simulink model "WInd_Blade_Simulation"  (R2022b)
settings: Solver=VariableStepAuto  StartTime=0.0  StopTime=10.0  RelTol=1e-3
settings Model: Creator=jayesh sunil gurav  LastModifiedBy=Amol Gavit
settings DebuggingCC: UnconnectedInputMsg=warning  UnconnectedOutputMsg=warning  UnconnectedLineMsg=warning
settings ModelReferenceCC: EnableRefExpFcnMdlSchedulingChecks=on
settings RTWCC: DLArmComputeVersion=19.05

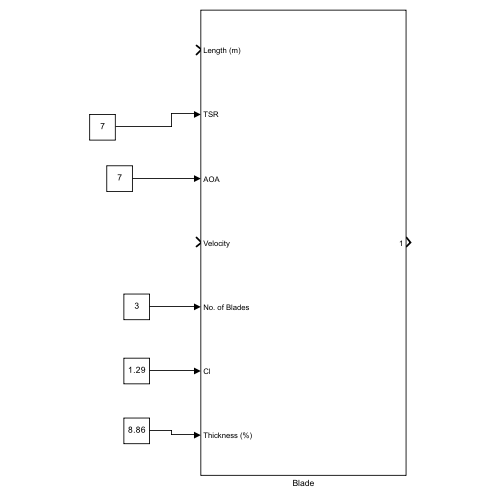
[thumbnail: Simulink's stored preview of the top-level diagram]
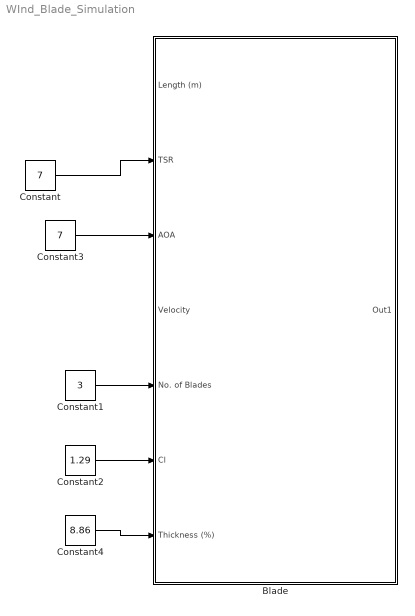
== system WInd_Blade_Simulation ==
  Blade : Subsystem
  Constant : Constant  Value=7
  Constant1 : Constant  Value=3
  Constant2 : Constant  Value=1.29
  Constant3 : Constant  Value=7
  Constant4 : Constant  Value=8.86
  wires:
  Constant/1 -> Blade/2(TSR)
  Constant1/1 -> Blade/5(No. of Blades)
  Constant2/1 -> Blade/6(Cl)
  Constant3/1 -> Blade/3(AOA)
  Constant4/1 -> Blade/7(Thickness (%))

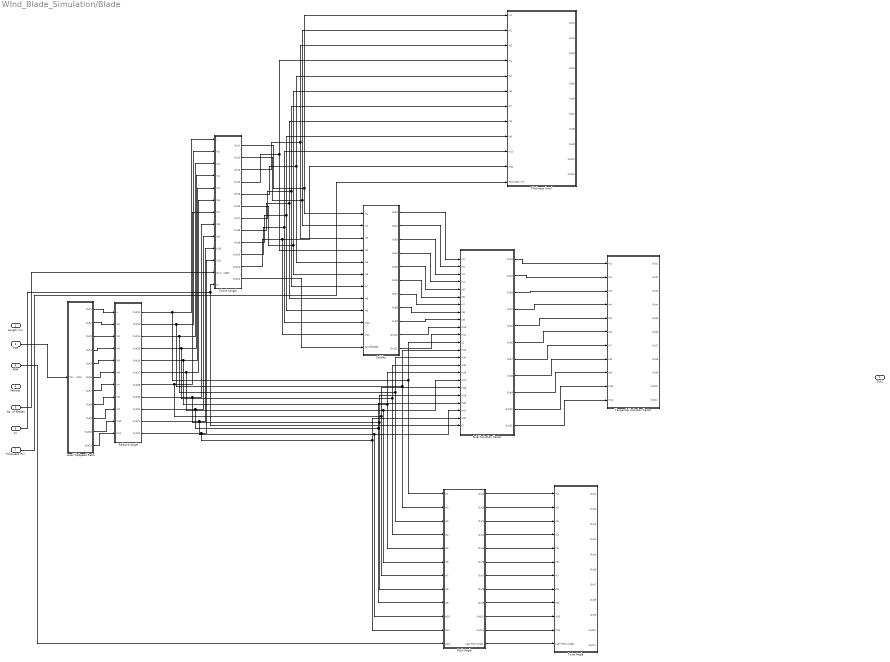
== system WInd_Blade_Simulation/Blade ==
  Length (m) : Inport
  TSR : Inport  Port=2
  AOA : Inport  Port=3
  Velocity : Inport  Port=4
  No. of Blades : Inport  Port=5
  Cl : Inport  Port=6
  Thickness (%) : Inport  Port=7
  Axial Induction Factor : Subsystem
  Chord Length : Subsystem
  Local TipSpeed Ratio : Subsystem
  Pitch Angle : Subsystem
  Relative Angle : Subsystem
  Solidity : Subsystem
  Tangential Induction Factor : Subsystem
  Thickness (mm) : Subsystem
  Twist Angle : Subsystem
  Out1 : Outport
  wires:
  TSR/1 -> Local TipSpeed Ratio/1(Tip Speed ratio)
  Local TipSpeed Ratio/1(Out1) -> Relative Angle/1(u)
  Local TipSpeed Ratio/2(Out2) -> Relative Angle/2(In2)
  Local TipSpeed Ratio/11(Out11) -> Relative Angle/11(In11)
  Local TipSpeed Ratio/10(Out10) -> Relative Angle/10(In10)
  Local TipSpeed Ratio/9(Out9) -> Relative Angle/9(In9)
  Local TipSpeed Ratio/8(Out8) -> Relative Angle/8(In8)
  Local TipSpeed Ratio/7(Out7) -> Relative Angle/7(In7)
  Local TipSpeed Ratio/6(Out6) -> Relative Angle/6(In6)
  Local TipSpeed Ratio/5(Out5) -> Relative Angle/5(In5)
  Local TipSpeed Ratio/4(Out4) -> Relative Angle/4(In4)
  Local TipSpeed Ratio/3(Out3) -> Relative Angle/3(In3)
  Relative Angle/1(Out12) -> Pitch Angle/1(In1), Axial Induction Factor/12(12), Chord Length/1(1)
  Relative Angle/2(Out13) -> Pitch Angle/2(In2), Axial Induction Factor/13(In13), Chord Length/2(In2)
  Relative Angle/3(Out14) -> Pitch Angle/3(In3), Axial Induction Factor/14(In14), Chord Length/3(In3)
  Relative Angle/4(Out15) -> Pitch Angle/4(In4), Axial Induction Factor/15(In15), Chord Length/4(In4)
  Relative Angle/5(Out16) -> Pitch Angle/5(In5), Axial Induction Factor/16(In16), Chord Length/5(In5)
  Relative Angle/6(Out17) -> Pitch Angle/6(In6), Axial Induction Factor/17(In17), Chord Length/6(In6)
  Relative Angle/7(Out18) -> Pitch Angle/7(In7), Axial Induction Factor/18(In18), Chord Length/7(In7)
  Relative Angle/8(Out19) -> Pitch Angle/8(In8), Axial Induction Factor/19(In19), Chord Length/8(In8)
  Relative Angle/9(Out20) -> Pitch Angle/9(In9), Axial Induction Factor/20(In20), Chord Length/9(In9)
  Relative Angle/10(Out21) -> Pitch Angle/10(In10), Axial Induction Factor/21(In21), Chord Length/10(In10)
  Relative Angle/11(Out22) -> Pitch Angle/11(In11), Axial Induction Factor/22(In22), Chord Length/11(In11)
  No. of Blades/1 -> Chord Length/12(No of Blades)
  Cl/1 -> Chord Length/13(Cl), Axial Induction Factor/23(Cl)
  Chord Length/2(Out2) -> Thickness (mm)/2(In2), Solidity/2(In2)
  Chord Length/3(Out3) -> Solidity/3(In3), Thickness (mm)/3(In3)
  Chord Length/4(Out4) -> Solidity/4(In4), Thickness (mm)/4(In4)
  Chord Length/5(Out5) -> Solidity/5(In5), Thickness (mm)/5(In5)
  Chord Length/6(Out6) -> Solidity/6(In6), Thickness (mm)/6(In6)
  Chord Length/7(Out7) -> Solidity/7(In7), Thickness (mm)/7(In7)
  Chord Length/8(Out8) -> Solidity/8(In8), Thickness (mm)/8(In8)
  Chord Length/9(Out9) -> Solidity/9(In9), Thickness (mm)/9(In9)
  Chord Length/10(Out10) -> Solidity/10(In10), Thickness (mm)/10(In12)
  Chord Length/11(Out11) -> Solidity/11(In11), Thickness (mm)/11(In10)
  Chord Length/12(Out12) -> Solidity/12(No of Blades)
  Solidity/1(Out1) -> Axial Induction Factor/1(In1)
  Solidity/2(Out2) -> Axial Induction Factor/2(In2)
  Solidity/3(Out3) -> Axial Induction Factor/3(In3)
  Solidity/4(Out4) -> Axial Induction Factor/4(In4)
  Solidity/5(Out5) -> Axial Induction Factor/5(In5)
  Solidity/6(Out6) -> Axial Induction Factor/6(In6)
  Solidity/7(Out7) -> Axial Induction Factor/7(In7)
  Solidity/8(Out8) -> Axial Induction Factor/8(In8)
  Solidity/9(Out9) -> Axial Induction Factor/9(In9)
  Solidity/10(Out10) -> Axial Induction Factor/10(In10)
  Solidity/11(Out11) -> Axial Induction Factor/11(In11)
  Axial Induction Factor/1(Out1) -> Tangential Induction Factor/1(In1)
  Axial Induction Factor/2(Out2) -> Tangential Induction Factor/2(In2)
  Axial Induction Factor/3(Out3) -> Tangential Induction Factor/3(In3)
  Axial Induction Factor/4(Out4) -> Tangential Induction Factor/4(In4)
  Axial Induction Factor/5(Out5) -> Tangential Induction Factor/5(In5)
  Axial Induction Factor/6(Out6) -> Tangential Induction Factor/6(In6)
  Axial Induction Factor/7(Out7) -> Tangential Induction Factor/7(In7)
  Axial Induction Factor/8(Out8) -> Tangential Induction Factor/8(In8)
  Axial Induction Factor/9(Out9) -> Tangential Induction Factor/9(In9)
  Axial Induction Factor/10(Out10) -> Tangential Induction Factor/10(In10)
  Axial Induction Factor/11(Out11) -> Tangential Induction Factor/11(In11)
  AOA/1 -> Pitch Angle/12(AOA)
  Pitch Angle/1(Out1) -> Twist Angle/1(In1)
  Pitch Angle/2(Out3) -> Twist Angle/2(In2)
  Pitch Angle/3(Out2) -> Twist Angle/3(In3)
  Pitch Angle/4(Out4) -> Twist Angle/4(In4)
  Pitch Angle/5(Out5) -> Twist Angle/5(In5)
  Pitch Angle/6(Out6) -> Twist Angle/6(In6)
  Pitch Angle/7(Out7) -> Twist Angle/7(In7)
  Pitch Angle/8(Out8) -> Twist Angle/8(In8)
  Pitch Angle/9(Out9) -> Twist Angle/9(In9)
  Pitch Angle/10(Out10) -> Twist Angle/10(In10)
  Pitch Angle/11(Out11) -> Twist Angle/11(In11)
  Pitch Angle/12(Last Pitch angle) -> Twist Angle/12(Last Pitch Anlge)
  Chord Length/1(Out1) -> Thickness (mm)/1(In1), Solidity/1(In1)
  Thickness (%)/1 -> Thickness (mm)/12(Thickness (%))

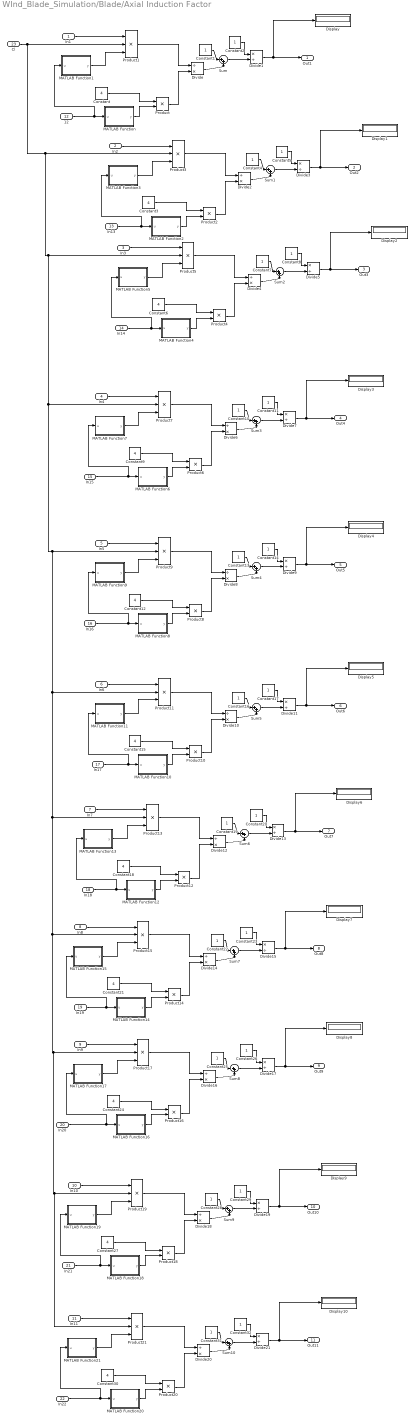
== system WInd_Blade_Simulation/Blade/Axial Induction Factor ==
  In1 : Inport
  In2 : Inport  Port=2
  In3 : Inport  Port=3
  In4 : Inport  Port=4
  In5 : Inport  Port=5
  In6 : Inport  Port=6
  In7 : Inport  Port=7
  In8 : Inport  Port=8
  In9 : Inport  Port=9
  In10 : Inport  Port=10
  In11 : Inport  Port=11
  12 : Inport  Port=12
  In13 : Inport  Port=13
  In14 : Inport  Port=14
  In15 : Inport  Port=15
  In16 : Inport  Port=16
  In17 : Inport  Port=17
  In18 : Inport  Port=18
  In19 : Inport  Port=19
  In20 : Inport  Port=20
  In21 : Inport  Port=21
  In22 : Inport  Port=22
  Cl : Inport  Port=23
  Constant{,3,6,9,12,15,18,21,24,27,30} (11 alike) : Constant  Value=4
  Constant{1..2,4..5,7..8,10..11,13..14,16..17,19..20,22..23,25..26,28..29,31..32} (22 alike) : Constant
  Display{,1..10} (11 alike) : Display
  Divide{,2,4,6,8,10,12,14,16,18,20} (11 alike) : Product  Inputs=/*
  Divide{1,3,5,7,9,11,13,15,17,19,21} (11 alike) : Product  Inputs=*/
  MATLAB Function : MATLAB Function  TreatAsAtomicUnit=on
  MATLAB Function1 : MATLAB Function  TreatAsAtomicUnit=on
  MATLAB Function10 : MATLAB Function  TreatAsAtomicUnit=on
  MATLAB Function11 : MATLAB Function  TreatAsAtomicUnit=on
  MATLAB Function12 : MATLAB Function  TreatAsAtomicUnit=on
  MATLAB Function13 : MATLAB Function  TreatAsAtomicUnit=on
  MATLAB Function14 : MATLAB Function  TreatAsAtomicUnit=on
  MATLAB Function15 : MATLAB Function  TreatAsAtomicUnit=on
  MATLAB Function16 : MATLAB Function  TreatAsAtomicUnit=on
  MATLAB Function17 : MATLAB Function  TreatAsAtomicUnit=on
  MATLAB Function18 : MATLAB Function  TreatAsAtomicUnit=on
  MATLAB Function19 : MATLAB Function  TreatAsAtomicUnit=on
  MATLAB Function2 : MATLAB Function  TreatAsAtomicUnit=on
  MATLAB Function20 : MATLAB Function  TreatAsAtomicUnit=on
  MATLAB Function21 : MATLAB Function  TreatAsAtomicUnit=on
  MATLAB Function3 : MATLAB Function  TreatAsAtomicUnit=on
  MATLAB Function4 : MATLAB Function  TreatAsAtomicUnit=on
  MATLAB Function5 : MATLAB Function  TreatAsAtomicUnit=on
  MATLAB Function6 : MATLAB Function  TreatAsAtomicUnit=on
  MATLAB Function7 : MATLAB Function  TreatAsAtomicUnit=on
  MATLAB Function8 : MATLAB Function  TreatAsAtomicUnit=on
  MATLAB Function9 : MATLAB Function  TreatAsAtomicUnit=on
  Product{,2,4,6,8,10,12,14,16,18,20} (11 alike) : Product
  Product{1,3,5,7,9,11,13,15,17,19,21} (11 alike) : Product  Inputs=3
  Sum{,1..10} (11 alike) : Sum  Inputs=|++
  Out1 : Outport
  Out2 : Outport  Port=2
  Out3 : Outport  Port=3
  Out4 : Outport  Port=4
  Out5 : Outport  Port=5
  Out6 : Outport  Port=6
  Out7 : Outport  Port=7
  Out8 : Outport  Port=8
  Out9 : Outport  Port=9
  Out10 : Outport  Port=10
  Out11 : Outport  Port=11
  wires:
  Constant/1 -> Product/1
  12/1 -> MATLAB Function1/1(u), MATLAB Function/1(u)
  MATLAB Function/1(y) -> Product/2
  In1/1 -> Product1/1
  MATLAB Function1/1(y) -> Product1/3
  Product1/1 -> Divide/1
  Product/1 -> Divide/2
  Constant1/1 -> Sum/1
  Divide/1 -> Sum/2
  Sum/1 -> Divide1/2
  Constant2/1 -> Divide1/1
  Divide1/1 -> Display/1, Out1/1
  In13/1 -> MATLAB Function2/1(u), MATLAB Function3/1(u)
  Sum1/1 -> Divide3/2
  MATLAB Function3/1(y) -> Product3/3
  Divide2/1 -> Sum1/2
  Divide3/1 -> Display1/1, Out2/1
  Product3/1 -> Divide2/1
  In2/1 -> Product3/1
  MATLAB Function2/1(y) -> Product2/2
  Constant4/1 -> Sum1/1
  Constant3/1 -> Product2/1
  Constant5/1 -> Divide3/1
  Product2/1 -> Divide2/2
  In14/1 -> MATLAB Function5/1(u), MATLAB Function4/1(u)
  Sum2/1 -> Divide5/2
  MATLAB Function5/1(y) -> Product5/3
  Divide4/1 -> Sum2/2
  Divide5/1 -> Display2/1, Out3/1
  Product5/1 -> Divide4/1
  In3/1 -> Product5/1
  MATLAB Function4/1(y) -> Product4/2
  Constant7/1 -> Sum2/1
  Constant6/1 -> Product4/1
  Constant8/1 -> Divide5/1
  Product4/1 -> Divide4/2
  In15/1 -> MATLAB Function7/1(u), MATLAB Function6/1(u)
  Sum3/1 -> Divide7/2
  MATLAB Function7/1(y) -> Product7/3
  Divide6/1 -> Sum3/2
  Divide7/1 -> Display3/1, Out4/1
  Product7/1 -> Divide6/1
  In4/1 -> Product7/1
  MATLAB Function6/1(y) -> Product6/2
  Constant10/1 -> Sum3/1
  Constant9/1 -> Product6/1
  Constant11/1 -> Divide7/1
  Product6/1 -> Divide6/2
  In16/1 -> MATLAB Function9/1(u), MATLAB Function8/1(u)
  Sum4/1 -> Divide9/2
  MATLAB Function9/1(y) -> Product9/3
  Divide8/1 -> Sum4/2
  Divide9/1 -> Display4/1, Out5/1
  Product9/1 -> Divide8/1
  In5/1 -> Product9/1
  MATLAB Function8/1(y) -> Product8/2
  Constant13/1 -> Sum4/1
  Constant12/1 -> Product8/1
  Constant14/1 -> Divide9/1
  Product8/1 -> Divide8/2
  In17/1 -> MATLAB Function11/1(u), MATLAB Function10/1(u)
  Sum5/1 -> Divide11/2
  MATLAB Function11/1(y) -> Product11/3
  Divide10/1 -> Sum5/2
  Divide11/1 -> Display5/1, Out6/1
  Product11/1 -> Divide10/1
  In6/1 -> Product11/1
  MATLAB Function10/1(y) -> Product10/2
  Constant16/1 -> Sum5/1
  Constant15/1 -> Product10/1
  Constant17/1 -> Divide11/1
  Product10/1 -> Divide10/2
  In18/1 -> MATLAB Function13/1(u), MATLAB Function12/1(u)
  Sum6/1 -> Divide13/2
  MATLAB Function13/1(y) -> Product13/3
  Divide12/1 -> Sum6/2
  Divide13/1 -> Display6/1, Out7/1
  Product13/1 -> Divide12/1
  In7/1 -> Product13/1
  MATLAB Function12/1(y) -> Product12/2
  Constant19/1 -> Sum6/1
  Constant18/1 -> Product12/1
  Constant20/1 -> Divide13/1
  Product12/1 -> Divide12/2
  In19/1 -> MATLAB Function14/1(u), MATLAB Function15/1(u)
  Sum7/1 -> Divide15/2
  MATLAB Function15/1(y) -> Product15/3
  Divide14/1 -> Sum7/2
  Divide15/1 -> Display7/1, Out8/1
  Product15/1 -> Divide14/1
  In8/1 -> Product15/1
  MATLAB Function14/1(y) -> Product14/2
  Constant22/1 -> Sum7/1
  Constant21/1 -> Product14/1
  Constant23/1 -> Divide15/1
  Product14/1 -> Divide14/2
  In20/1 -> MATLAB Function17/1(u), MATLAB Function16/1(u)
  Sum8/1 -> Divide17/2
  MATLAB Function17/1(y) -> Product17/3
  Divide16/1 -> Sum8/2
  Divide17/1 -> Display8/1, Out9/1
  Product17/1 -> Divide16/1
  In9/1 -> Product17/1
  MATLAB Function16/1(y) -> Product16/2
  Constant25/1 -> Sum8/1
  Constant24/1 -> Product16/1
  Constant26/1 -> Divide17/1
  Product16/1 -> Divide16/2
  In21/1 -> MATLAB Function19/1(u), MATLAB Function18/1(u)
  Sum9/1 -> Divide19/2
  MATLAB Function19/1(y) -> Product19/3
  Divide18/1 -> Sum9/2
  Divide19/1 -> Display9/1, Out10/1
  Product19/1 -> Divide18/1
  In10/1 -> Product19/1
  MATLAB Function18/1(y) -> Product18/2
  Constant28/1 -> Sum9/1
  Constant27/1 -> Product18/1
  Constant29/1 -> Divide19/1
  Product18/1 -> Divide18/2
  In22/1 -> MATLAB Function21/1(u), MATLAB Function20/1(u)
  Sum10/1 -> Divide21/2
  MATLAB Function21/1(y) -> Product21/3
  Divide20/1 -> Sum10/2
  Divide21/1 -> Display10/1, Out11/1
  Product21/1 -> Divide20/1
  In11/1 -> Product21/1
  Cl/1 -> Product3/2, Product5/2, Product21/2, Product19/2, Product17/2, Product15/2, Product13/2, Product11/2, Product9/2, Product7/2, Product1/2
  MATLAB Function20/1(y) -> Product20/2
  Constant31/1 -> Sum10/1
  Constant30/1 -> Product20/1
  Constant32/1 -> Divide21/1
  Product20/1 -> Divide20/2

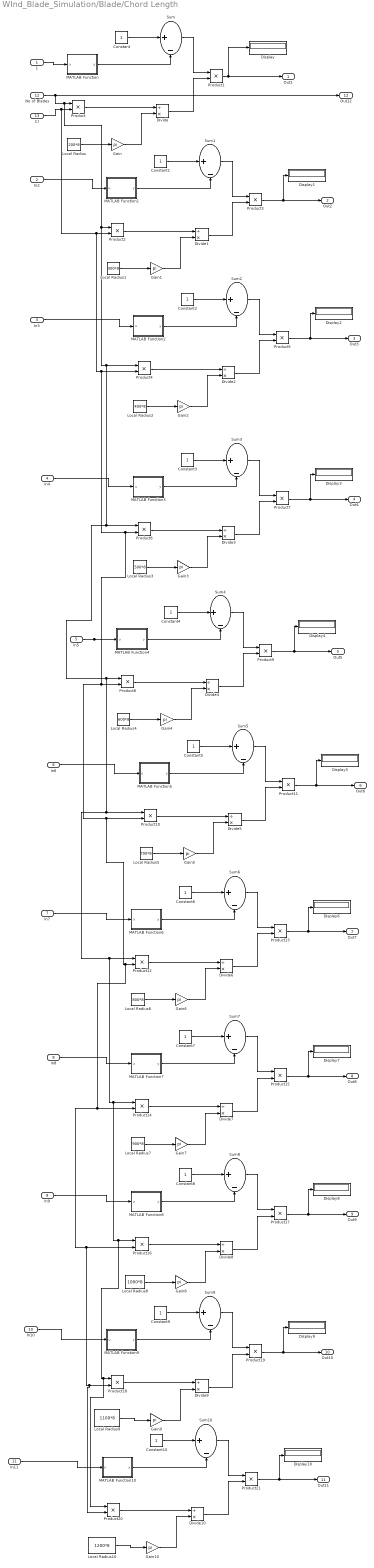
== system WInd_Blade_Simulation/Blade/Chord Length ==
  1 : Inport
  In2 : Inport  Port=2
  In3 : Inport  Port=3
  In4 : Inport  Port=4
  In5 : Inport  Port=5
  In6 : Inport  Port=6
  In7 : Inport  Port=7
  In8 : Inport  Port=8
  In9 : Inport  Port=9
  In10 : Inport  Port=10
  In11 : Inport  Port=11
  No of Blades : Inport  Port=12
  Cl : Inport  Port=13
  Constant{,1..10} (11 alike) : Constant
  Display{,1..10} (11 alike) : Display
  Divide{,1..10} (11 alike) : Product  Inputs=/*
  Gain{,1..10} (11 alike) : Gain  Gain=pi
  Local Radius : Constant  Value=200*8
  Local Radius1 : Constant  Value=300*8
  Local Radius10 : Constant  Value=1200*8
  Local Radius2 : Constant  Value=400*8
  Local Radius3 : Constant  Value=500*8
  Local Radius4 : Constant  Value=600*8
  Local Radius5 : Constant  Value=700*8
  Local Radius6 : Constant  Value=800*8
  Local Radius7 : Constant  Value=900*8
  Local Radius8 : Constant  Value=1000*8
  Local Radius9 : Constant  Value=1100*8
  MATLAB Function : MATLAB Function  TreatAsAtomicUnit=on
  MATLAB Function1 : MATLAB Function  TreatAsAtomicUnit=on
  MATLAB Function10 : MATLAB Function  TreatAsAtomicUnit=on
  MATLAB Function2 : MATLAB Function  TreatAsAtomicUnit=on
  MATLAB Function3 : MATLAB Function  TreatAsAtomicUnit=on
  MATLAB Function4 : MATLAB Function  TreatAsAtomicUnit=on
  MATLAB Function5 : MATLAB Function  TreatAsAtomicUnit=on
  MATLAB Function6 : MATLAB Function  TreatAsAtomicUnit=on
  MATLAB Function7 : MATLAB Function  TreatAsAtomicUnit=on
  MATLAB Function8 : MATLAB Function  TreatAsAtomicUnit=on
  MATLAB Function9 : MATLAB Function  TreatAsAtomicUnit=on
  Product{,1..21} (22 alike) : Product
  Sum{,1..10} (11 alike) : Sum  Inputs=|+-
  Out1 : Outport
  Out2 : Outport  Port=2
  Out3 : Outport  Port=3
  Out4 : Outport  Port=4
  Out5 : Outport  Port=5
  Out6 : Outport  Port=6
  Out7 : Outport  Port=7
  Out8 : Outport  Port=8
  Out9 : Outport  Port=9
  Out10 : Outport  Port=10
  Out11 : Outport  Port=11
  Out12 : Outport  Port=12
  wires:
  Local Radius/1 -> Gain/1
  Gain/1 -> Divide/2
  Product/1 -> Divide/1
  Divide/1 -> Product1/2
  1/1 -> MATLAB Function/1(u)
  Constant/1 -> Sum/1
  MATLAB Function/1(y) -> Sum/2
  Sum/1 -> Product1/1
  Product1/1 -> Display/1, Out1/1
  Product3/1 -> Display1/1, Out2/1
  Divide1/1 -> Product3/2
  In2/1 -> MATLAB Function1/1(u)
  Sum1/1 -> Product3/1
  MATLAB Function1/1(y) -> Sum1/2
  Gain1/1 -> Divide1/2
  Constant1/1 -> Sum1/1
  Product2/1 -> Divide1/1
  Local Radius1/1 -> Gain1/1
  Product4/1 -> Divide2/1
  MATLAB Function2/1(y) -> Sum2/2
  Divide2/1 -> Product5/2
  Gain2/1 -> Divide2/2
  Product5/1 -> Display2/1, Out3/1
  In3/1 -> MATLAB Function2/1(u)
  Sum2/1 -> Product5/1
  Local Radius2/1 -> Gain2/1
  Constant2/1 -> Sum2/1
  Product6/1 -> Divide3/1
  MATLAB Function3/1(y) -> Sum3/2
  Divide3/1 -> Product7/2
  Gain3/1 -> Divide3/2
  Product7/1 -> Display3/1, Out4/1
  In4/1 -> MATLAB Function3/1(u)
  Sum3/1 -> Product7/1
  Local Radius3/1 -> Gain3/1
  Constant3/1 -> Sum3/1
  Product8/1 -> Divide4/1
  MATLAB Function4/1(y) -> Sum4/2
  Divide4/1 -> Product9/2
  Gain4/1 -> Divide4/2
  Product9/1 -> Display4/1, Out5/1
  In5/1 -> MATLAB Function4/1(u)
  Sum4/1 -> Product9/1
  Local Radius4/1 -> Gain4/1
  Constant4/1 -> Sum4/1
  Constant5/1 -> Sum5/1
  Sum5/1 -> Product11/1
  Local Radius5/1 -> Gain5/1
  Product11/1 -> Display5/1, Out6/1
  Divide5/1 -> Product11/2
  In6/1 -> MATLAB Function5/1(u)
  Product10/1 -> Divide5/1
  Gain5/1 -> Divide5/2
  MATLAB Function5/1(y) -> Sum5/2
  Constant6/1 -> Sum6/1
  Sum6/1 -> Product13/1
  Local Radius6/1 -> Gain6/1
  Product13/1 -> Display6/1, Out7/1
  Divide6/1 -> Product13/2
  In7/1 -> MATLAB Function6/1(u)
  Product12/1 -> Divide6/1
  Gain6/1 -> Divide6/2
  MATLAB Function6/1(y) -> Sum6/2
  Constant7/1 -> Sum7/1
  Sum7/1 -> Product15/1
  Local Radius7/1 -> Gain7/1
  Product15/1 -> Display7/1, Out8/1
  Divide7/1 -> Product15/2
  In8/1 -> MATLAB Function7/1(u)
  Product14/1 -> Divide7/1
  Gain7/1 -> Divide7/2
  MATLAB Function7/1(y) -> Sum7/2
  Constant8/1 -> Sum8/1
  Sum8/1 -> Product17/1
  Local Radius8/1 -> Gain8/1
  Product17/1 -> Display8/1, Out9/1
  Divide8/1 -> Product17/2
  In9/1 -> MATLAB Function8/1(u)
  Product16/1 -> Divide8/1
  Gain8/1 -> Divide8/2
  MATLAB Function8/1(y) -> Sum8/2
  Constant9/1 -> Sum9/1
  Sum9/1 -> Product19/1
  Local Radius9/1 -> Gain9/1
  Product19/1 -> Display9/1, Out10/1
  Divide9/1 -> Product19/2
  In10/1 -> MATLAB Function9/1(u)
  Product18/1 -> Divide9/1
  Gain9/1 -> Divide9/2
  MATLAB Function9/1(y) -> Sum9/2
  Constant10/1 -> Sum10/1
  Sum10/1 -> Product21/1
  No of Blades/1 -> Product2/1, Product6/1, Product8/1, Product10/1, Product20/1, Product18/1, Product16/1, Product14/1, Product12/1, Product4/1, Product/1, Out12/1
  Local Radius10/1 -> Gain10/1
  Product21/1 -> Display10/1, Out11/1
  Divide10/1 -> Product21/2
  In11/1 -> MATLAB Function10/1(u)
  Product20/1 -> Divide10/1
  Cl/1 -> Product4/2, Product8/2, Product14/2, Product20/2, Product18/2, Product16/2, Product12/2, Product10/2, Product6/2, Product2/2, Product/2
  Gain10/1 -> Divide10/2
  MATLAB Function10/1(y) -> Sum10/2

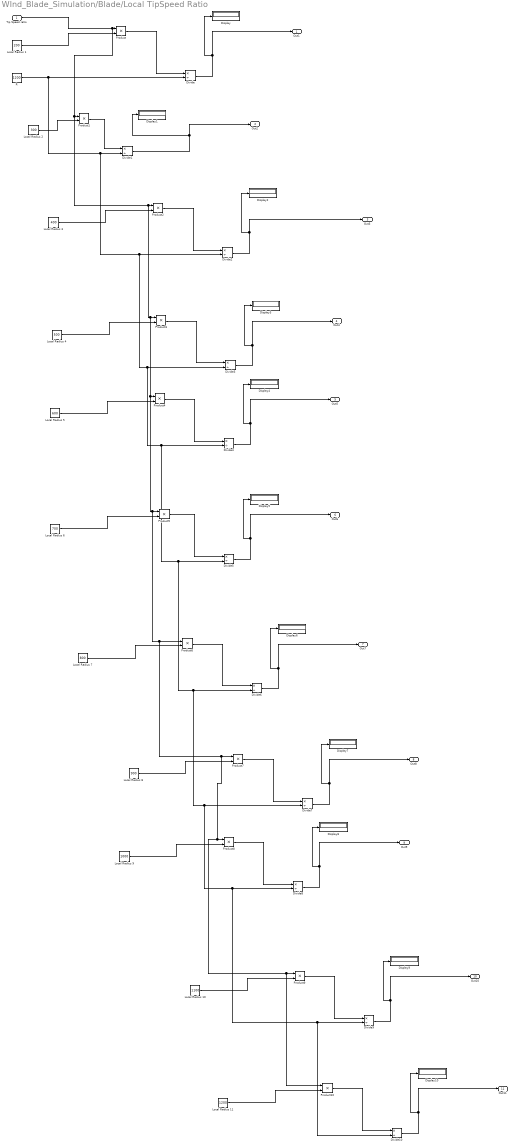
== system WInd_Blade_Simulation/Blade/Local TipSpeed Ratio ==
  Tip Speed ratio : Inport
  Display{,1..10} (11 alike) : Display
  Divide{,1..10} (11 alike) : Product  Inputs=*/
  Local Radius 1 : Constant  Value=200
  Local Radius 10 : Constant  Value=1100
  Local Radius 11 : Constant  Value=1200
  Local Radius 2 : Constant  Value=300
  Local Radius 3 : Constant  Value=400
  Local Radius 4 : Constant  Value=500
  Local Radius 5 : Constant  Value=600
  Local Radius 6 : Constant  Value=700
  Local Radius 7 : Constant  Value=800
  Local Radius 8 : Constant  Value=900
  Local Radius 9 : Constant  Value=1000
  Product{,1..10} (11 alike) : Product
  R : Constant  Value=1200
  Out1 : Outport
  Out2 : Outport  Port=2
  Out3 : Outport  Port=3
  Out4 : Outport  Port=4
  Out5 : Outport  Port=5
  Out6 : Outport  Port=6
  Out7 : Outport  Port=7
  Out8 : Outport  Port=8
  Out9 : Outport  Port=9
  Out10 : Outport  Port=10
  Out11 : Outport  Port=11
  wires:
  Product/1 -> Divide/1
  Divide/1 -> Display/1, Out1/1
  Local Radius 1/1 -> Product/2
  Divide1/1 -> Display1/1, Out2/1
  Local Radius 2/1 -> Product1/2
  Product1/1 -> Divide1/1
  Local Radius 3/1 -> Product2/2
  Product2/1 -> Divide2/1
  Divide2/1 -> Out3/1, Display2/1
  Product3/1 -> Divide3/1
  Divide3/1 -> Out4/1, Display3/1
  Local Radius 4/1 -> Product3/2
  Local Radius 5/1 -> Product4/2
  Product4/1 -> Divide4/1
  Divide4/1 -> Out5/1, Display4/1
  Local Radius 6/1 -> Product5/2
  Product5/1 -> Divide5/1
  Divide5/1 -> Out6/1, Display5/1
  Local Radius 7/1 -> Product6/2
  Product6/1 -> Divide6/1
  Divide6/1 -> Out7/1, Display6/1
  Local Radius 8/1 -> Product7/2
  Product7/1 -> Divide7/1
  Divide7/1 -> Out8/1, Display7/1
  Local Radius 9/1 -> Product8/2
  Product8/1 -> Divide8/1
  Divide8/1 -> Out9/1, Display8/1
  Local Radius 10/1 -> Product9/2
  Product9/1 -> Divide9/1
  Divide9/1 -> Out10/1, Display9/1
  R/1 -> Divide5/2, Divide10/2, Divide9/2, Divide8/2, Divide7/2, Divide6/2, Divide4/2, Divide3/2, Divide2/2, Divide1/2, Divide/2
  Local Radius 11/1 -> Product10/2
  Product10/1 -> Divide10/1
  Divide10/1 -> Out11/1, Display10/1
  Tip Speed ratio/1 -> Product8/1, Product10/1, Product9/1, Product7/1, Product6/1, Product5/1, Product4/1, Product3/1, Product2/1, Product1/1, Product/1

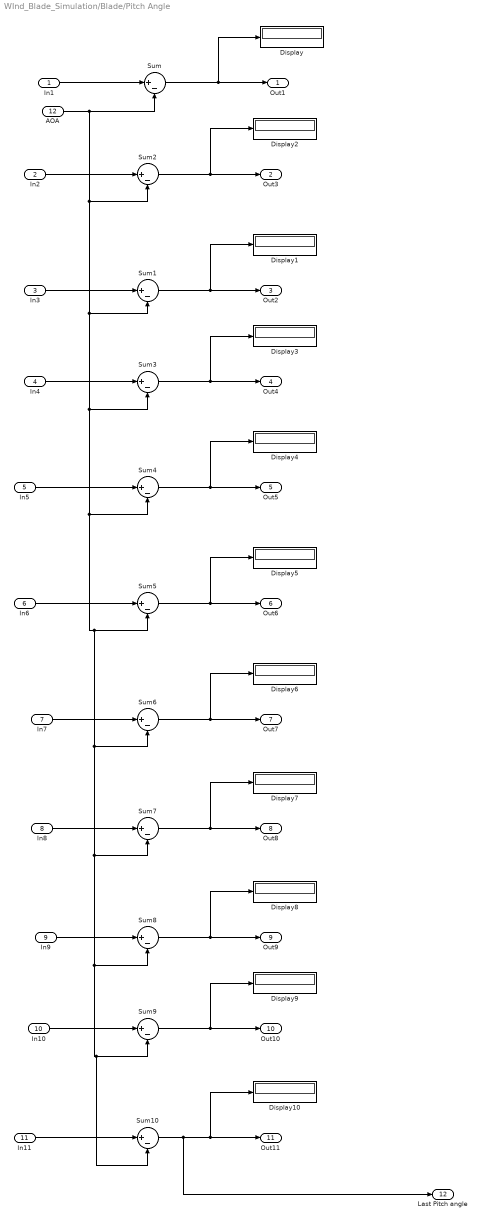
== system WInd_Blade_Simulation/Blade/Pitch Angle ==
  In1 : Inport
  In2 : Inport  Port=2
  In3 : Inport  Port=3
  In4 : Inport  Port=4
  In5 : Inport  Port=5
  In6 : Inport  Port=6
  In7 : Inport  Port=7
  In8 : Inport  Port=8
  In9 : Inport  Port=9
  In10 : Inport  Port=10
  In11 : Inport  Port=11
  AOA : Inport  Port=12
  Display{,1..10} (11 alike) : Display
  Sum{,1..10} (11 alike) : Sum  Inputs=|+-
  Out1 : Outport
  Out3 : Outport  Port=2
  Out2 : Outport  Port=3
  Out4 : Outport  Port=4
  Out5 : Outport  Port=5
  Out6 : Outport  Port=6
  Out7 : Outport  Port=7
  Out8 : Outport  Port=8
  Out9 : Outport  Port=9
  Out10 : Outport  Port=10
  Out11 : Outport  Port=11
  Last Pitch angle : Outport  Port=12
  wires:
  In1/1 -> Sum/1
  Sum/1 -> Display/1, Out1/1
  Sum2/1 -> Display2/1, Out3/1
  In2/1 -> Sum2/1
  Sum1/1 -> Display1/1, Out2/1
  In3/1 -> Sum1/1
  Sum3/1 -> Display3/1, Out4/1
  In4/1 -> Sum3/1
  Sum4/1 -> Display4/1, Out5/1
  In5/1 -> Sum4/1
  Sum5/1 -> Display5/1, Out6/1
  In6/1 -> Sum5/1
  Sum6/1 -> Display6/1, Out7/1
  In7/1 -> Sum6/1
  Sum7/1 -> Display7/1, Out8/1
  In8/1 -> Sum7/1
  Sum8/1 -> Display8/1, Out9/1
  In9/1 -> Sum8/1
  Sum9/1 -> Display9/1, Out10/1
  In10/1 -> Sum9/1
  Sum10/1 -> Last Pitch angle/1, Display10/1, Out11/1
  AOA/1 -> Sum2/2, Sum1/2, Sum3/2, Sum6/2, Sum8/2, Sum10/2, Sum9/2, Sum7/2, Sum5/2, Sum4/2, Sum/2
  In11/1 -> Sum10/1

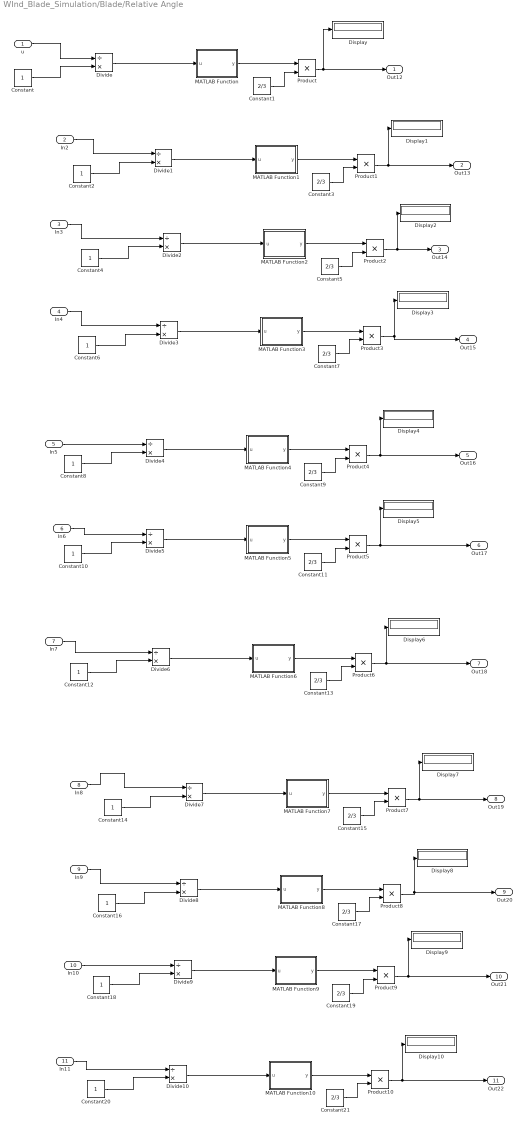
== system WInd_Blade_Simulation/Blade/Relative Angle ==
  u : Inport
  In2 : Inport  Port=2
  In3 : Inport  Port=3
  In4 : Inport  Port=4
  In5 : Inport  Port=5
  In6 : Inport  Port=6
  In7 : Inport  Port=7
  In8 : Inport  Port=8
  In9 : Inport  Port=9
  In10 : Inport  Port=10
  In11 : Inport  Port=11
  Constant{,2,4,6,8,10,12,14,16,18,20} (11 alike) : Constant
  Constant{1,3,5,7,9,11,13,15,17,19,21} (11 alike) : Constant  Value=2/3
  Display{,1..10} (11 alike) : Display
  Divide{,1..10} (11 alike) : Product  Inputs=/*
  MATLAB Function : MATLAB Function  TreatAsAtomicUnit=on
  MATLAB Function1 : MATLAB Function  TreatAsAtomicUnit=on
  MATLAB Function10 : MATLAB Function  TreatAsAtomicUnit=on
  MATLAB Function2 : MATLAB Function  TreatAsAtomicUnit=on
  MATLAB Function3 : MATLAB Function  TreatAsAtomicUnit=on
  MATLAB Function4 : MATLAB Function  TreatAsAtomicUnit=on
  MATLAB Function5 : MATLAB Function  TreatAsAtomicUnit=on
  MATLAB Function6 : MATLAB Function  TreatAsAtomicUnit=on
  MATLAB Function7 : MATLAB Function  TreatAsAtomicUnit=on
  MATLAB Function8 : MATLAB Function  TreatAsAtomicUnit=on
  MATLAB Function9 : MATLAB Function  TreatAsAtomicUnit=on
  Product{,1..10} (11 alike) : Product
  Out12 : Outport
  Out13 : Outport  Port=2
  Out14 : Outport  Port=3
  Out15 : Outport  Port=4
  Out16 : Outport  Port=5
  Out17 : Outport  Port=6
  Out18 : Outport  Port=7
  Out19 : Outport  Port=8
  Out20 : Outport  Port=9
  Out21 : Outport  Port=10
  Out22 : Outport  Port=11
  wires:
  u/1 -> Divide/1
  Constant/1 -> Divide/2
  Divide/1 -> MATLAB Function/1(u)
  MATLAB Function/1(y) -> Product/1
  Constant1/1 -> Product/2
  Product/1 -> Display/1, Out12/1
  In2/1 -> Divide1/1
  Product1/1 -> Display1/1, Out13/1
  MATLAB Function1/1(y) -> Product1/1
  Constant3/1 -> Product1/2
  Divide1/1 -> MATLAB Function1/1(u)
  Constant2/1 -> Divide1/2
  In3/1 -> Divide2/1
  Constant4/1 -> Divide2/2
  Product2/1 -> Display2/1, Out14/1
  MATLAB Function2/1(y) -> Product2/1
  Constant5/1 -> Product2/2
  Divide2/1 -> MATLAB Function2/1(u)
  In4/1 -> Divide3/1
  Constant6/1 -> Divide3/2
  Product3/1 -> Display3/1, Out15/1
  MATLAB Function3/1(y) -> Product3/1
  Constant7/1 -> Product3/2
  Divide3/1 -> MATLAB Function3/1(u)
  In5/1 -> Divide4/1
  Constant8/1 -> Divide4/2
  Product4/1 -> Display4/1, Out16/1
  MATLAB Function4/1(y) -> Product4/1
  Constant9/1 -> Product4/2
  Divide4/1 -> MATLAB Function4/1(u)
  In6/1 -> Divide5/1
  Constant10/1 -> Divide5/2
  Product5/1 -> Display5/1, Out17/1
  MATLAB Function5/1(y) -> Product5/1
  Constant11/1 -> Product5/2
  Divide5/1 -> MATLAB Function5/1(u)
  In7/1 -> Divide6/1
  Constant12/1 -> Divide6/2
  Product6/1 -> Display6/1, Out18/1
  MATLAB Function6/1(y) -> Product6/1
  Constant13/1 -> Product6/2
  Divide6/1 -> MATLAB Function6/1(u)
  In8/1 -> Divide7/1
  Constant14/1 -> Divide7/2
  Product7/1 -> Display7/1, Out19/1
  MATLAB Function7/1(y) -> Product7/1
  Constant15/1 -> Product7/2
  Divide7/1 -> MATLAB Function7/1(u)
  In9/1 -> Divide8/1
  Constant16/1 -> Divide8/2
  Product8/1 -> Display8/1, Out20/1
  MATLAB Function8/1(y) -> Product8/1
  Constant17/1 -> Product8/2
  Divide8/1 -> MATLAB Function8/1(u)
  In10/1 -> Divide9/1
  Constant18/1 -> Divide9/2
  Product9/1 -> Display9/1, Out21/1
  MATLAB Function9/1(y) -> Product9/1
  Constant19/1 -> Product9/2
  Divide9/1 -> MATLAB Function9/1(u)
  In11/1 -> Divide10/1
  Constant20/1 -> Divide10/2
  Product10/1 -> Display10/1, Out22/1
  MATLAB Function10/1(y) -> Product10/1
  Constant21/1 -> Product10/2
  Divide10/1 -> MATLAB Function10/1(u)

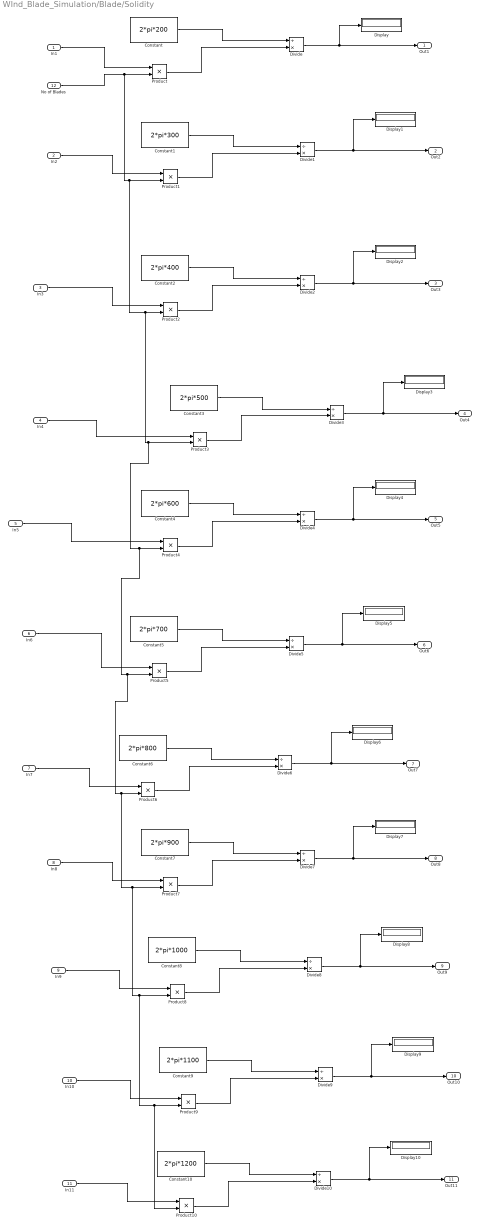
== system WInd_Blade_Simulation/Blade/Solidity ==
  In1 : Inport
  In2 : Inport  Port=2
  In3 : Inport  Port=3
  In4 : Inport  Port=4
  In5 : Inport  Port=5
  In6 : Inport  Port=6
  In7 : Inport  Port=7
  In8 : Inport  Port=8
  In9 : Inport  Port=9
  In10 : Inport  Port=10
  In11 : Inport  Port=11
  No of Blades : Inport  Port=12
  Constant : Constant  Value=2*pi*200
  Constant1 : Constant  Value=2*pi*300
  Constant10 : Constant  Value=2*pi*1200
  Constant2 : Constant  Value=2*pi*400
  Constant3 : Constant  Value=2*pi*500
  Constant4 : Constant  Value=2*pi*600
  Constant5 : Constant  Value=2*pi*700
  Constant6 : Constant  Value=2*pi*800
  Constant7 : Constant  Value=2*pi*900
  Constant8 : Constant  Value=2*pi*1000
  Constant9 : Constant  Value=2*pi*1100
  Display{,1..10} (11 alike) : Display
  Divide{,1..10} (11 alike) : Product  Inputs=/*
  Product{,1..10} (11 alike) : Product
  Out1 : Outport
  Out2 : Outport  Port=2
  Out3 : Outport  Port=3
  Out4 : Outport  Port=4
  Out5 : Outport  Port=5
  Out6 : Outport  Port=6
  Out7 : Outport  Port=7
  Out8 : Outport  Port=8
  Out9 : Outport  Port=9
  Out10 : Outport  Port=10
  Out11 : Outport  Port=11
  wires:
  In1/1 -> Product/1
  Product/1 -> Divide/2
  Constant/1 -> Divide/1
  Divide/1 -> Display/1, Out1/1
  Product1/1 -> Divide1/2
  Divide1/1 -> Display1/1, Out2/1
  Constant1/1 -> Divide1/1
  In2/1 -> Product1/1
  In3/1 -> Product2/1
  Constant2/1 -> Divide2/1
  Divide2/1 -> Display2/1, Out3/1
  Product2/1 -> Divide2/2
  In4/1 -> Product3/1
  Constant3/1 -> Divide3/1
  Divide3/1 -> Display3/1, Out4/1
  Product3/1 -> Divide3/2
  In5/1 -> Product4/1
  Constant4/1 -> Divide4/1
  Divide4/1 -> Display4/1, Out5/1
  Product4/1 -> Divide4/2
  In6/1 -> Product5/1
  Constant5/1 -> Divide5/1
  Divide5/1 -> Display5/1, Out6/1
  Product5/1 -> Divide5/2
  In7/1 -> Product6/1
  Constant6/1 -> Divide6/1
  Divide6/1 -> Display6/1, Out7/1
  Product6/1 -> Divide6/2
  In8/1 -> Product7/1
  Constant7/1 -> Divide7/1
  Divide7/1 -> Display7/1, Out8/1
  Product7/1 -> Divide7/2
  In9/1 -> Product8/1
  Constant8/1 -> Divide8/1
  Divide8/1 -> Display8/1, Out9/1
  Product8/1 -> Divide8/2
  In10/1 -> Product9/1
  Constant9/1 -> Divide9/1
  Divide9/1 -> Display9/1, Out10/1
  Product9/1 -> Divide9/2
  In11/1 -> Product10/1
  No of Blades/1 -> Product10/2, Product9/2, Product8/2, Product7/2, Product6/2, Product5/2, Product4/2, Product3/2, Product2/2, Product1/2, Product/2
  Constant10/1 -> Divide10/1
  Divide10/1 -> Display10/1, Out11/1
  Product10/1 -> Divide10/2

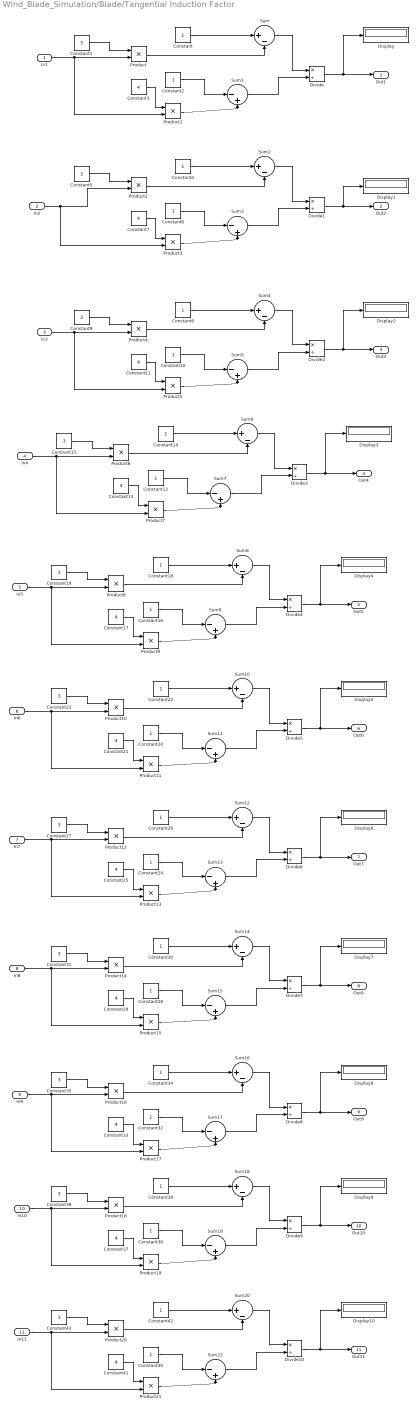
== system WInd_Blade_Simulation/Blade/Tangential Induction Factor ==
  In1 : Inport
  In2 : Inport  Port=2
  In3 : Inport  Port=3
  In4 : Inport  Port=4
  In5 : Inport  Port=5
  In6 : Inport  Port=6
  In7 : Inport  Port=7
  In8 : Inport  Port=8
  In9 : Inport  Port=9
  In10 : Inport  Port=10
  In11 : Inport  Port=11
  Constant{,2,4,6,8,10,12,14,16,18,20,22,24,26,28,30,32,34,36,38,40,42} (22 alike) : Constant
  Constant{1,5,9,15,19,23,27,31,35,39,43} (11 alike) : Constant  Value=3
  Constant{3,7,11,13,17,21,25,29,33,37,41} (11 alike) : Constant  Value=4
  Display{,1..10} (11 alike) : Display
  Divide{,1..10} (11 alike) : Product  Inputs=*/
  Product{,1..21} (22 alike) : Product
  Sum{,2,4,6,8,10,12,14,16,18,20} (11 alike) : Sum  Inputs=|+-
  Sum{1,3,5,7,9,11,13,15,17,19,21} (11 alike) : Sum  Inputs=|-+
  Out1 : Outport
  Out2 : Outport  Port=2
  Out3 : Outport  Port=3
  Out4 : Outport  Port=4
  Out5 : Outport  Port=5
  Out6 : Outport  Port=6
  Out7 : Outport  Port=7
  Out8 : Outport  Port=8
  Out9 : Outport  Port=9
  Out10 : Outport  Port=10
  Out11 : Outport  Port=11
  wires:
  Constant/1 -> Sum/1
  Product/1 -> Sum/2
  Constant3/1 -> Product1/1
  Constant1/1 -> Product/1
  In1/1 -> Product1/2, Product/2
  Constant2/1 -> Sum1/1
  Product1/1 -> Sum1/2
  Sum/1 -> Divide/1
  Sum1/1 -> Divide/2
  Divide/1 -> Out1/1, Display/1
  Constant5/1 -> Product2/1
  Product2/1 -> Sum2/2
  Sum3/1 -> Divide1/2
  Constant4/1 -> Sum2/1
  Product3/1 -> Sum3/2
  Constant6/1 -> Sum3/1
  Sum2/1 -> Divide1/1
  Divide1/1 -> Out2/1, Display1/1
  Constant7/1 -> Product3/1
  Constant9/1 -> Product4/1
  In3/1 -> Product5/2, Product4/2
  Product4/1 -> Sum4/2
  Sum5/1 -> Divide2/2
  Constant8/1 -> Sum4/1
  Product5/1 -> Sum5/2
  Constant10/1 -> Sum5/1
  Sum4/1 -> Divide2/1
  Divide2/1 -> Out3/1, Display2/1
  Constant11/1 -> Product5/1
  In2/1 -> Product3/2, Product2/2
  Constant13/1 -> Product7/1
  Sum6/1 -> Divide3/1
  Constant14/1 -> Sum6/1
  Product7/1 -> Sum7/2
  Sum7/1 -> Divide3/2
  Constant12/1 -> Sum7/1
  Constant15/1 -> Product6/1
  Product6/1 -> Sum6/2
  Divide3/1 -> Out4/1, Display3/1
  In4/1 -> Product7/2, Product6/2
  Constant17/1 -> Product9/1
  Sum8/1 -> Divide4/1
  Constant18/1 -> Sum8/1
  Product9/1 -> Sum9/2
  Sum9/1 -> Divide4/2
  Constant16/1 -> Sum9/1
  Constant19/1 -> Product8/1
  Product8/1 -> Sum8/2
  Divide4/1 -> Out5/1, Display4/1
  In5/1 -> Product9/2, Product8/2
  Constant21/1 -> Product11/1
  Sum10/1 -> Divide5/1
  Constant22/1 -> Sum10/1
  Product11/1 -> Sum11/2
  Sum11/1 -> Divide5/2
  Constant20/1 -> Sum11/1
  Constant23/1 -> Product10/1
  Product10/1 -> Sum10/2
  Divide5/1 -> Out6/1, Display5/1
  In6/1 -> Product11/2, Product10/2
  Constant25/1 -> Product13/1
  Sum12/1 -> Divide6/1
  Constant26/1 -> Sum12/1
  Product13/1 -> Sum13/2
  Sum13/1 -> Divide6/2
  Constant24/1 -> Sum13/1
  Constant27/1 -> Product12/1
  Product12/1 -> Sum12/2
  Divide6/1 -> Out7/1, Display6/1
  In7/1 -> Product13/2, Product12/2
  Constant29/1 -> Product15/1
  Sum14/1 -> Divide7/1
  Constant30/1 -> Sum14/1
  Product15/1 -> Sum15/2
  Sum15/1 -> Divide7/2
  Constant28/1 -> Sum15/1
  Constant31/1 -> Product14/1
  Product14/1 -> Sum14/2
  Divide7/1 -> Out8/1, Display7/1
  In8/1 -> Product15/2, Product14/2
  Constant33/1 -> Product17/1
  Sum16/1 -> Divide8/1
  Constant34/1 -> Sum16/1
  Product17/1 -> Sum17/2
  Sum17/1 -> Divide8/2
  Constant32/1 -> Sum17/1
  Constant35/1 -> Product16/1
  Product16/1 -> Sum16/2
  Divide8/1 -> Out9/1, Display8/1
  In9/1 -> Product17/2, Product16/2
  Constant37/1 -> Product19/1
  Sum18/1 -> Divide9/1
  Constant38/1 -> Sum18/1
  Product19/1 -> Sum19/2
  Sum19/1 -> Divide9/2
  Constant36/1 -> Sum19/1
  Constant39/1 -> Product18/1
  Product18/1 -> Sum18/2
  Divide9/1 -> Out10/1, Display9/1
  In10/1 -> Product19/2, Product18/2
  Constant41/1 -> Product21/1
  Sum20/1 -> Divide10/1
  Constant42/1 -> Sum20/1
  Product21/1 -> Sum21/2
  Sum21/1 -> Divide10/2
  Constant40/1 -> Sum21/1
  Constant43/1 -> Product20/1
  Product20/1 -> Sum20/2
  Divide10/1 -> Out11/1, Display10/1
  In11/1 -> Product21/2, Product20/2

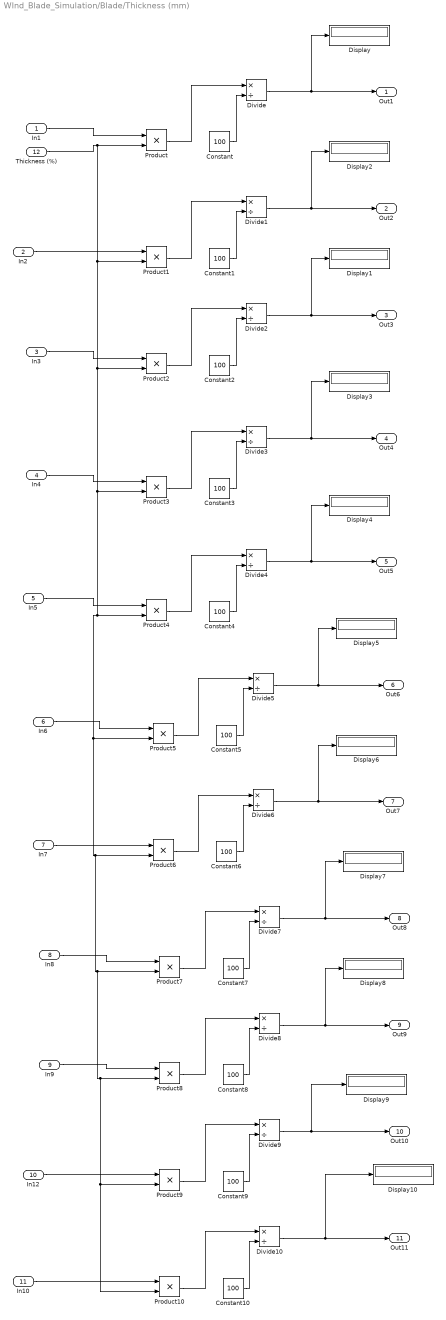
== system WInd_Blade_Simulation/Blade/Thickness (mm) ==
  In1 : Inport
  In2 : Inport  Port=2
  In3 : Inport  Port=3
  In4 : Inport  Port=4
  In5 : Inport  Port=5
  In6 : Inport  Port=6
  In7 : Inport  Port=7
  In8 : Inport  Port=8
  In9 : Inport  Port=9
  In12 : Inport  Port=10
  In10 : Inport  Port=11
  Thickness (%) : Inport  Port=12
  Constant{,1..10} (11 alike) : Constant  Value=100
  Display{,1..10} (11 alike) : Display
  Divide{,1..10} (11 alike) : Product  Inputs=*/
  Product{,1..10} (11 alike) : Product
  Out1 : Outport
  Out2 : Outport  Port=2
  Out3 : Outport  Port=3
  Out4 : Outport  Port=4
  Out5 : Outport  Port=5
  Out6 : Outport  Port=6
  Out7 : Outport  Port=7
  Out8 : Outport  Port=8
  Out9 : Outport  Port=9
  Out10 : Outport  Port=10
  Out11 : Outport  Port=11
  wires:
  In1/1 -> Product/1
  Product/1 -> Divide/1
  Constant/1 -> Divide/2
  Divide/1 -> Display/1, Out1/1
  Divide1/1 -> Display2/1, Out2/1
  Product1/1 -> Divide1/1
  Constant1/1 -> Divide1/2
  In2/1 -> Product1/1
  Divide2/1 -> Display1/1, Out3/1
  Product2/1 -> Divide2/1
  Constant2/1 -> Divide2/2
  In3/1 -> Product2/1
  Divide3/1 -> Display3/1, Out4/1
  Product3/1 -> Divide3/1
  Constant3/1 -> Divide3/2
  In4/1 -> Product3/1
  Divide4/1 -> Display4/1, Out5/1
  Product4/1 -> Divide4/1
  Constant4/1 -> Divide4/2
  In5/1 -> Product4/1
  Divide5/1 -> Display5/1, Out6/1
  Product5/1 -> Divide5/1
  Constant5/1 -> Divide5/2
  In6/1 -> Product5/1
  Divide6/1 -> Display6/1, Out7/1
  Product6/1 -> Divide6/1
  Constant6/1 -> Divide6/2
  In7/1 -> Product6/1
  Divide7/1 -> Display7/1, Out8/1
  Product7/1 -> Divide7/1
  Constant7/1 -> Divide7/2
  In8/1 -> Product7/1
  Divide8/1 -> Display8/1, Out9/1
  Product8/1 -> Divide8/1
  Constant8/1 -> Divide8/2
  In9/1 -> Product8/1
  Constant9/1 -> Divide9/2
  Product9/1 -> Divide9/1
  Divide9/1 -> Display9/1, Out10/1
  In12/1 -> Product9/1
  Constant10/1 -> Divide10/2
  Product10/1 -> Divide10/1
  Divide10/1 -> Display10/1, Out11/1
  In10/1 -> Product10/1
  Thickness (%)/1 -> Product10/2, Product9/2, Product8/2, Product7/2, Product6/2, Product5/2, Product4/2, Product3/2, Product2/2, Product1/2, Product/2

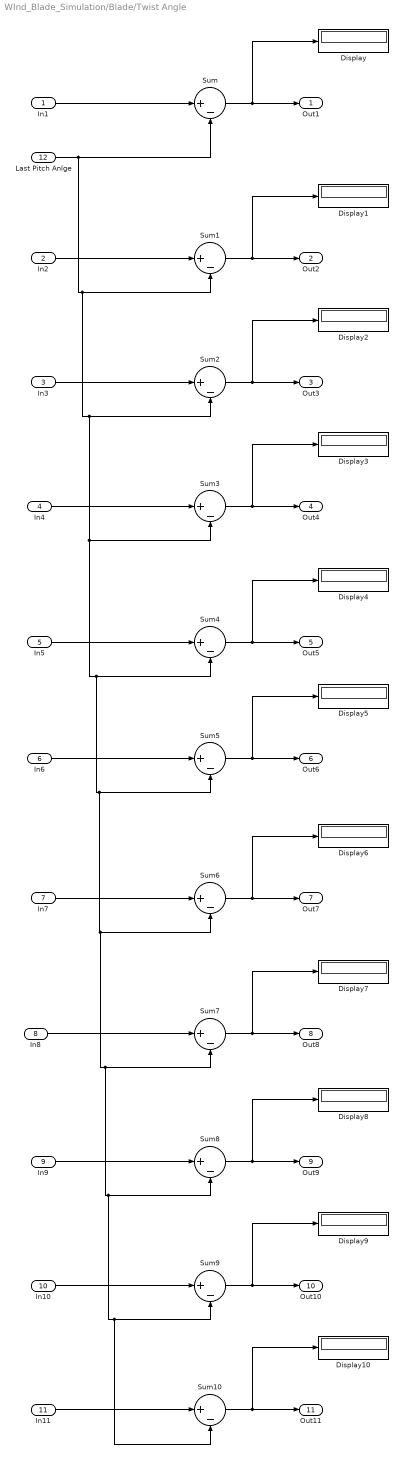
== system WInd_Blade_Simulation/Blade/Twist Angle ==
  In1 : Inport
  In2 : Inport  Port=2
  In3 : Inport  Port=3
  In4 : Inport  Port=4
  In5 : Inport  Port=5
  In6 : Inport  Port=6
  In7 : Inport  Port=7
  In8 : Inport  Port=8
  In9 : Inport  Port=9
  In10 : Inport  Port=10
  In11 : Inport  Port=11
  Last Pitch Anlge : Inport  Port=12
  Display{,1..10} (11 alike) : Display
  Sum{,1..10} (11 alike) : Sum  Inputs=|+-
  Out1 : Outport
  Out2 : Outport  Port=2
  Out3 : Outport  Port=3
  Out4 : Outport  Port=4
  Out5 : Outport  Port=5
  Out6 : Outport  Port=6
  Out7 : Outport  Port=7
  Out8 : Outport  Port=8
  Out9 : Outport  Port=9
  Out10 : Outport  Port=10
  Out11 : Outport  Port=11
  wires:
  In1/1 -> Sum/1
  Sum/1 -> Display/1, Out1/1
  Sum1/1 -> Display1/1, Out2/1
  In2/1 -> Sum1/1
  Sum2/1 -> Display2/1, Out3/1
  In3/1 -> Sum2/1
  Sum3/1 -> Display3/1, Out4/1
  In4/1 -> Sum3/1
  Sum4/1 -> Display4/1, Out5/1
  In5/1 -> Sum4/1
  Sum5/1 -> Display5/1, Out6/1
  In6/1 -> Sum5/1
  Sum6/1 -> Display6/1, Out7/1
  In7/1 -> Sum6/1
  Sum7/1 -> Display7/1, Out8/1
  In8/1 -> Sum7/1
  Sum8/1 -> Display8/1, Out9/1
  In9/1 -> Sum8/1
  Sum9/1 -> Display9/1, Out10/1
  In10/1 -> Sum9/1
  Sum10/1 -> Display10/1, Out11/1
  In11/1 -> Sum10/1
  Last Pitch Anlge/1 -> Sum10/2, Sum9/2, Sum8/2, Sum7/2, Sum6/2, Sum5/2, Sum4/2, Sum3/2, Sum2/2, Sum1/2, Sum/2

== matlab function WInd_Blade_Simulation/Blade/Chord Length/MATLAB Function3 ==
  data: u input; y output
function y = fcn(u)

y =cosd(u);
end

== matlab function WInd_Blade_Simulation/Blade/Chord Length/MATLAB Function4 ==
  data: u input; y output
function y = fcn(u)

y =cosd(u);
end

== matlab function WInd_Blade_Simulation/Blade/Chord Length/MATLAB Function5 ==
  data: u input; y output
function y = fcn(u)

y =cosd(u);
end

== matlab function WInd_Blade_Simulation/Blade/Chord Length/MATLAB Function6 ==
  data: u input; y output
function y = fcn(u)

y =cosd(u);
end

== matlab function WInd_Blade_Simulation/Blade/Chord Length/MATLAB Function7 ==
  data: u input; y output
function y = fcn(u)

y =cosd(u);
end

== matlab function WInd_Blade_Simulation/Blade/Relative Angle/MATLAB Function ==
  data: u input; y output
function y = fcn(u)

y = atand(u);
end

== matlab function WInd_Blade_Simulation/Blade/Chord Length/MATLAB Function8 ==
  data: u input; y output
function y = fcn(u)

y =cosd(u);
end

== matlab function WInd_Blade_Simulation/Blade/Chord Length/MATLAB Function9 ==
  data: u input; y output
function y = fcn(u)

y =cosd(u);
end

== matlab function WInd_Blade_Simulation/Blade/Chord Length/MATLAB Function10 ==
  data: u input; y output
function y = fcn(u)

y =cosd(u);
end

== matlab function WInd_Blade_Simulation/Blade/Axial Induction Factor/MATLAB Function ==
  data: u input; y output
function y = fcn(u)

y =sind(u)^2;
end

== matlab function WInd_Blade_Simulation/Blade/Axial Induction Factor/MATLAB Function1 ==
  data: u input; y output
function y = fcn(u)

y =cosd(u);
end

== matlab function WInd_Blade_Simulation/Blade/Axial Induction Factor/MATLAB Function2 ==
  data: u input; y output
function y = fcn(u)

y =sind(u)^2;
end

== matlab function WInd_Blade_Simulation/Blade/Axial Induction Factor/MATLAB Function3 ==
  data: u input; y output
function y = fcn(u)

y =cosd(u);
end

== matlab function WInd_Blade_Simulation/Blade/Axial Induction Factor/MATLAB Function4 ==
  data: u input; y output
function y = fcn(u)

y =sind(u)^2;
end

== matlab function WInd_Blade_Simulation/Blade/Axial Induction Factor/MATLAB Function5 ==
  data: u input; y output
function y = fcn(u)

y =cosd(u);
end

== matlab function WInd_Blade_Simulation/Blade/Axial Induction Factor/MATLAB Function6 ==
  data: u input; y output
function y = fcn(u)

y =sind(u)^2;
end

== matlab function WInd_Blade_Simulation/Blade/Relative Angle/MATLAB Function2 ==
  data: u input; y output
function y = fcn(u)

y = atand(u);
end

== matlab function WInd_Blade_Simulation/Blade/Axial Induction Factor/MATLAB Function7 ==
  data: u input; y output
function y = fcn(u)

y =cosd(u);
end

== matlab function WInd_Blade_Simulation/Blade/Axial Induction Factor/MATLAB Function8 ==
  data: u input; y output
function y = fcn(u)

y =sind(u)^2;
end

== matlab function WInd_Blade_Simulation/Blade/Axial Induction Factor/MATLAB Function9 ==
  data: u input; y output
function y = fcn(u)

y =cosd(u);
end

== matlab function WInd_Blade_Simulation/Blade/Axial Induction Factor/MATLAB Function10 ==
  data: u input; y output
function y = fcn(u)

y =sind(u)^2;
end

== matlab function WInd_Blade_Simulation/Blade/Axial Induction Factor/MATLAB Function11 ==
  data: u input; y output
function y = fcn(u)

y =cosd(u);
end

== matlab function WInd_Blade_Simulation/Blade/Axial Induction Factor/MATLAB Function12 ==
  data: u input; y output
function y = fcn(u)

y =sind(u)^2;
end

== matlab function WInd_Blade_Simulation/Blade/Axial Induction Factor/MATLAB Function13 ==
  data: u input; y output
function y = fcn(u)

y =cosd(u);
end

== matlab function WInd_Blade_Simulation/Blade/Axial Induction Factor/MATLAB Function14 ==
  data: u input; y output
function y = fcn(u)

y =sind(u)^2;
end

== matlab function WInd_Blade_Simulation/Blade/Axial Induction Factor/MATLAB Function15 ==
  data: u input; y output
function y = fcn(u)

y =cosd(u);
end

== matlab function WInd_Blade_Simulation/Blade/Axial Induction Factor/MATLAB Function16 ==
  data: u input; y output
function y = fcn(u)

y =sind(u)^2;
end

== matlab function WInd_Blade_Simulation/Blade/Relative Angle/MATLAB Function3 ==
  data: u input; y output
function y = fcn(u)

y = atand(u);
end

== matlab function WInd_Blade_Simulation/Blade/Axial Induction Factor/MATLAB Function17 ==
  data: u input; y output
function y = fcn(u)

y =cosd(u);
end

== matlab function WInd_Blade_Simulation/Blade/Axial Induction Factor/MATLAB Function18 ==
  data: u input; y output
function y = fcn(u)

y =sind(u)^2;
end

== matlab function WInd_Blade_Simulation/Blade/Axial Induction Factor/MATLAB Function19 ==
  data: u input; y output
function y = fcn(u)

y =cosd(u);
end

== matlab function WInd_Blade_Simulation/Blade/Axial Induction Factor/MATLAB Function20 ==
  data: u input; y output
function y = fcn(u)

y =sind(u)^2;
end

== matlab function WInd_Blade_Simulation/Blade/Axial Induction Factor/MATLAB Function21 ==
  data: u input; y output
function y = fcn(u)

y =cosd(u);
end

== matlab function WInd_Blade_Simulation/Blade/Relative Angle/MATLAB Function4 ==
  data: u input; y output
function y = fcn(u)

y = atand(u);
end

== matlab function WInd_Blade_Simulation/Blade/Relative Angle/MATLAB Function5 ==
  data: u input; y output
function y = fcn(u)

y = atand(u);
end

== matlab function WInd_Blade_Simulation/Blade/Relative Angle/MATLAB Function6 ==
  data: u input; y output
function y = fcn(u)

y = atand(u);
end

== matlab function WInd_Blade_Simulation/Blade/Relative Angle/MATLAB Function7 ==
  data: u input; y output
function y = fcn(u)

y = atand(u);
end

== matlab function WInd_Blade_Simulation/Blade/Relative Angle/MATLAB Function8 ==
  data: u input; y output
function y = fcn(u)

y = atand(u);
end

== matlab function WInd_Blade_Simulation/Blade/Relative Angle/MATLAB Function1 ==
  data: u input; y output
function y = fcn(u)

y = atand(u);
end

== matlab function WInd_Blade_Simulation/Blade/Relative Angle/MATLAB Function9 ==
  data: u input; y output
function y = fcn(u)

y = atand(u);
end

== matlab function WInd_Blade_Simulation/Blade/Relative Angle/MATLAB Function10 ==
  data: u input; y output
function y = fcn(u)

y = atand(u);
end

== matlab function WInd_Blade_Simulation/Blade/Chord Length/MATLAB Function ==
  data: u input; y output
function y = fcn(u)

y =cosd(u);
end

== matlab function WInd_Blade_Simulation/Blade/Chord Length/MATLAB Function1 ==
  data: u input; y output
function y = fcn(u)

y =cosd(u);
end

== matlab function WInd_Blade_Simulation/Blade/Chord Length/MATLAB Function2 ==
  data: u input; y output
function y = fcn(u)

y =cosd(u);
end
